simulink model "Verifica_LQR_27042026"  (R2025b)
settings: Solver=VariableStepAuto  StartTime=0.0  StopTime=20.0  RelTol=1e-3
undefined symbols (not defined in the file): A, B, K_LQR_i, K_LQR_x, n, r
settings Model: Creator=salvo  LastModifiedBy=salvo

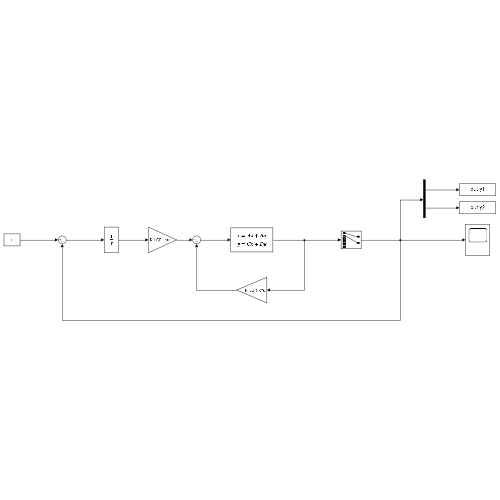
[thumbnail: Simulink's stored preview of the top-level diagram]
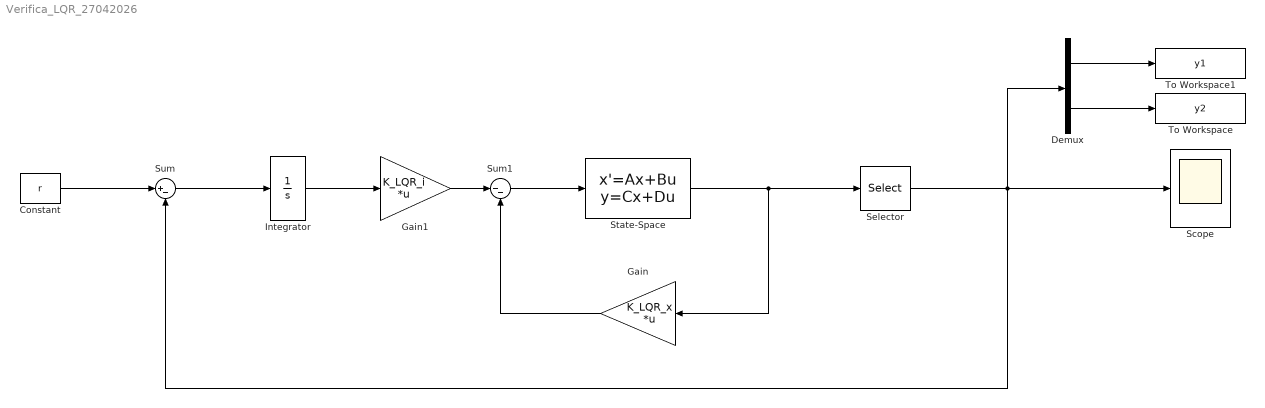
== system Verifica_LQR_27042026 ==
  Constant : Constant  Value=r
  Demux : Demux  Outputs=2
  Gain : Gain  Gain=K_LQR_x  Multiplication=Matrix(K*u)
  Gain1 : Gain  Gain=K_LQR_i  Multiplication=Matrix(K*u)
  Integrator : Integrator
  Scope : Scope
      settings: ActiveDisplayYMinimum=0.17614045657442728  ActiveDisplayYMaximum=0.34308216718089724
  Selector : Selector  InputPortWidth=6  IndexOptions=Index vector (dialog)  Indices=[1 2]  OutputSizes=1
  State-Space : StateSpace  A=A  B=B  C=eye(n)  D=zeros(6,2)  InitialCondition=0
  Sum : Sum  Inputs=|+-
  Sum1 : Sum  Inputs=|--
  To Workspace : ToWorkspace  VariableName=y2  SaveFormat=Timeseries  SampleTime=-1
  To Workspace1 : ToWorkspace  VariableName=y1  SaveFormat=Timeseries  SampleTime=-1
  wires:
  Gain1/1 -> Sum1/1
  Sum1/1 -> State-Space/1
  Gain/1 -> Sum1/2
  Integrator/1 -> Gain1/1
  Constant/1 -> Sum/1
  Sum/1 -> Integrator/1
  State-Space/1 -> Selector/1, Gain/1
  Selector/1 -> Demux/1, Sum/2, Scope/1
  Demux/2 -> To Workspace/1
  Demux/1 -> To Workspace1/1
